simulink model "simulacion_grua"  (R2021a)
settings: Solver=VariableStepAuto  StartTime=0.0  StopTime=20  RelTol=1e-3
values from neighbouring files (symbols this model uses):
  At = [0 0 1 0;0 0 0 1;0 0 -denp(2) 0; 0 -dena(3) 0 -dena(2)]    [modelo_grua_controles.m]
  Bt = [0;numa(2);nump(3);g_ktecho*numa(3)]    [modelo_grua_controles.m]
  Ctc = [1 0 0 0]    [modelo_grua_controles.m]
  K = Ks(1:4)    [modelo_grua_controles.m]
  K_lqr = Kss(1:4)    [modelo_grua_controles.m]
  Ki = -Ks(5)    [modelo_grua_controles.m]
  Ki_lqr = -Kss(5)    [modelo_grua_controles.m]
libraries: simulink x2
settings Model: Creator=Esteban Arias  LastModifiedBy=Esteban Arias
settings DataIOCC: ReturnWorkspaceOutputs=off

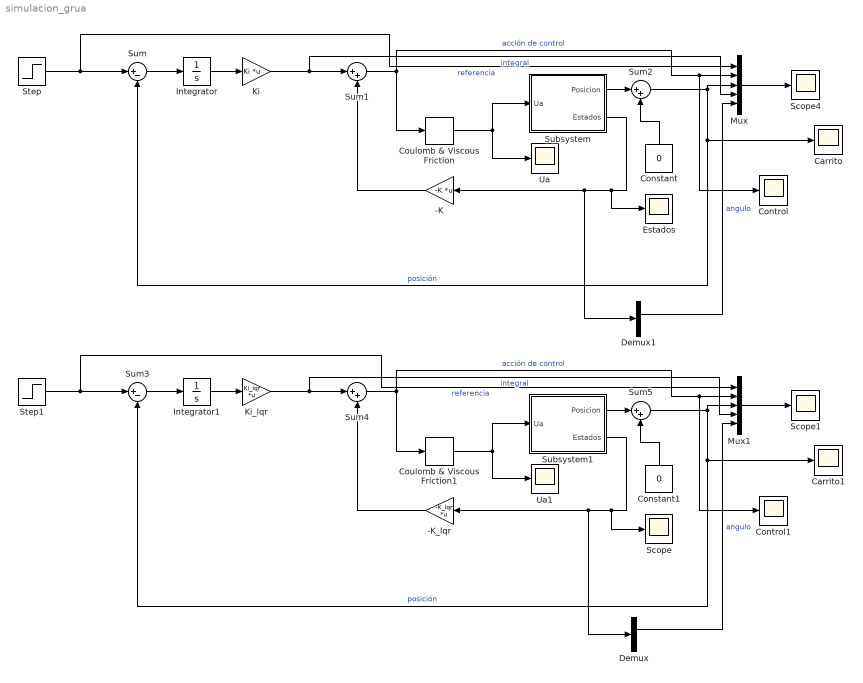
== system simulacion_grua ==
  -K : Gain  Gain=-K  Multiplication=Matrix(K*u)
  -K_lqr : Gain  Gain=-K_lqr  Multiplication=Matrix(K*u)
  Carrito : Scope
  Carrito1 : Scope
  Constant : Constant  Value=0
  Constant1 : Constant  Value=0
  Control : Scope
  Control1 : Scope
  Coulomb & Viscous Friction : simulink/Discontinuities/Coulomb & Viscous Friction  offset=[0.4]  gain=1
  Coulomb & Viscous Friction1 : simulink/Discontinuities/Coulomb & Viscous Friction  offset=[0.4]  gain=1
  Demux : Demux
  Demux1 : Demux
  Estados : Scope
  Integrator : Integrator
  Integrator1 : Integrator
  Ki : Gain  Gain=Ki  Multiplication=Matrix(K*u)
  Ki_lqr : Gain  Gain=Ki_lqr  Multiplication=Matrix(K*u)
  Mux : Mux  Inputs=5
  Mux1 : Mux  Inputs=5
  Scope : Scope
  Scope1 : Scope
  Scope4 : Scope
  Step : Step  Time=0  After=0.5  SampleTime=0
  Step1 : Step  Time=0  After=0.5  SampleTime=0
  Subsystem : Subsystem
  Subsystem1 : Subsystem
  Sum : Sum  Inputs=|+-
  Sum{1..2,4..5} (4 alike) : Sum  Inputs=|++
  Sum3 : Sum  Inputs=|+-
  Ua : Scope
  Ua1 : Scope
  wires:
  Step/1 -> Mux/1, Sum/1  "referencia"
  Sum/1 -> Integrator/1
  Integrator/1 -> Ki/1
  Ki/1 -> Mux/4, Sum1/1  "integral"
  Sum1/1 -> Control/1, Mux/2, Coulomb & Viscous Friction/1  "acción de control"
  -K/1 -> Sum1/2
  Coulomb & Viscous Friction/1 -> Ua/1, Subsystem/1(Ua)
  Subsystem/2(Estados) -> Estados/1, Demux1/1, -K/1
  Subsystem/1(Posicion) -> Sum2/1
  Sum2/1 -> Mux/3, Carrito/1, Sum/2  "posición"
  Mux/1 -> Scope4/1
  Constant/1 -> Sum2/2
  Constant1/1 -> Sum5/2
  Subsystem1/2(Estados) -> Scope/1, Demux/1, -K_lqr/1
  Coulomb & Viscous Friction1/1 -> Ua1/1, Subsystem1/1(Ua)
  -K_lqr/1 -> Sum4/2
  Subsystem1/1(Posicion) -> Sum5/1
  Sum5/1 -> Mux1/3, Carrito1/1, Sum3/2  "posición"
  Mux1/1 -> Scope1/1
  Sum4/1 -> Control1/1, Mux1/2, Coulomb & Viscous Friction1/1  "acción de control"
  Ki_lqr/1 -> Mux1/4, Sum4/1  "integral"
  Step1/1 -> Mux1/1, Sum3/1  "referencia"
  Sum3/1 -> Integrator1/1
  Integrator1/1 -> Ki_lqr/1
  Demux/2 -> Mux1/5  "angulo"
  Demux1/2 -> Mux/5  "angulo"

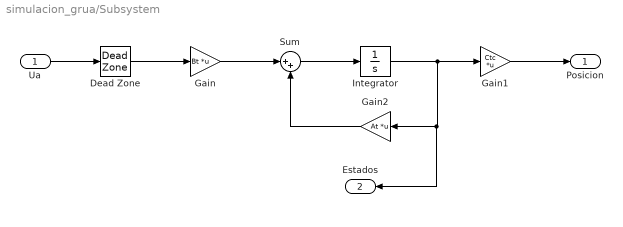
== system simulacion_grua/Subsystem ==
  Ua : Inport
  Dead Zone : DeadZone  UpperValue=0.6  SaturateOnIntegerOverflow=on
  Gain : Gain  Gain=Bt  Multiplication=Matrix(K*u)
  Gain1 : Gain  Gain=Ctc  Multiplication=Matrix(K*u)
  Gain2 : Gain  Gain=At  Multiplication=Matrix(K*u)
  Integrator : Integrator
  Sum : Sum  Inputs=|++
  Posicion : Outport
  Estados : Outport  Port=2
  wires:
  Gain/1 -> Sum/1
  Integrator/1 -> Estados/1, Gain2/1, Gain1/1
  Sum/1 -> Integrator/1
  Gain2/1 -> Sum/2
  Gain1/1 -> Posicion/1
  Dead Zone/1 -> Gain/1
  Ua/1 -> Dead Zone/1

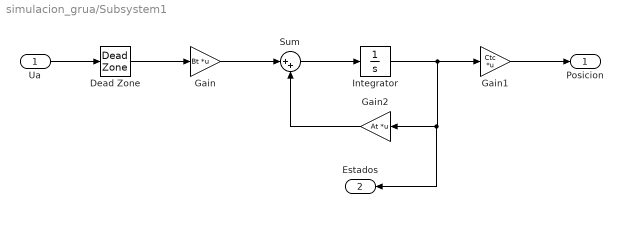
== system simulacion_grua/Subsystem1 ==
  Ua : Inport
  Dead Zone : DeadZone  UpperValue=0.6  SaturateOnIntegerOverflow=on
  Gain : Gain  Gain=Bt  Multiplication=Matrix(K*u)
  Gain1 : Gain  Gain=Ctc  Multiplication=Matrix(K*u)
  Gain2 : Gain  Gain=At  Multiplication=Matrix(K*u)
  Integrator : Integrator
  Sum : Sum  Inputs=|++
  Posicion : Outport
  Estados : Outport  Port=2
  wires:
  Gain/1 -> Sum/1
  Integrator/1 -> Estados/1, Gain2/1, Gain1/1
  Sum/1 -> Integrator/1
  Gain2/1 -> Sum/2
  Gain1/1 -> Posicion/1
  Dead Zone/1 -> Gain/1
  Ua/1 -> Dead Zone/1
